simulink model "cardio_v3"  (Simulink 7.4)
settings: Solver=ode45  StartTime=0.0  StopTime=100  RelTol=1e-3
settings Model: Creator=hp  LastModifiedBy=MXKana
settings DebuggingCC: SaveWithParameterizedLinksMsg=none

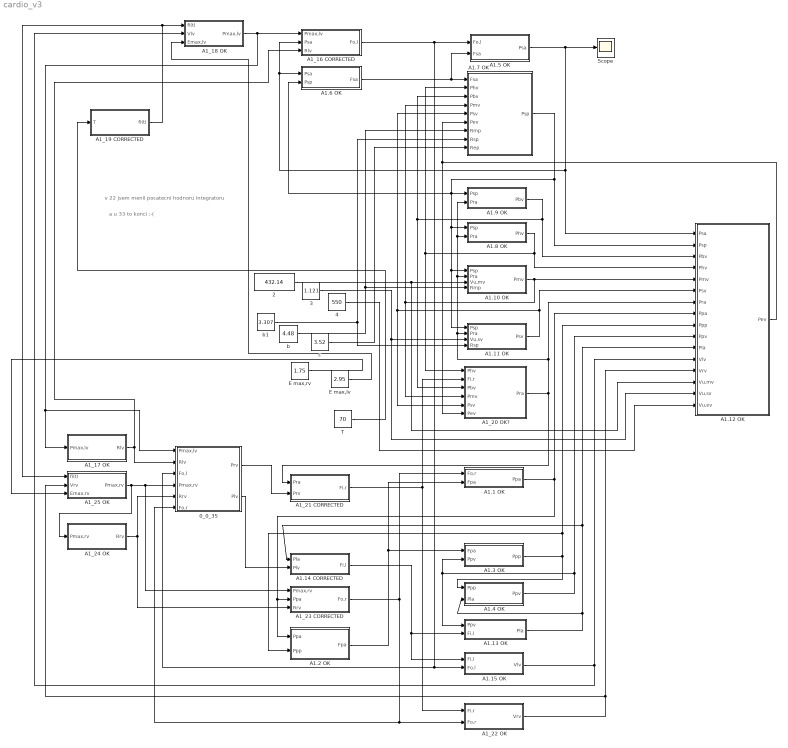
== system cardio_v3 ==
  note: v 22 jsem menil pocatecni hodnoru integratoru
  note: a u 33 to konci :-(
  0_0_35 : Subsystem
  2 : Constant  Value=432.14  OutDataType=sfix(16)  OutScaling=2^0
  3 : Constant  Value=1.121  OutDataType=sfix(16)  OutScaling=2^0
  4 : Constant  Value=550  OutDataType=sfix(16)  OutScaling=2^0
  A1.1 OK : Subsystem
  A1.10 OK : Subsystem
  A1.11 OK : Subsystem
  A1.12 OK : Subsystem
  A1.13 OK : Subsystem
  A1.14 CORRECTED : Subsystem
  A1.15 OK : Subsystem
  A1.2 OK : Subsystem
  A1.3 OK : Subsystem
  A1.4 OK : Subsystem
  A1.5 OK : Subsystem
  A1.6 OK : Subsystem
  A1.7 OK : Subsystem
  A1.8 OK : Subsystem
  A1.9 OK : Subsystem
  A1_16 CORRECTED : Subsystem
  A1_17 OK : Subsystem
  A1_18 OK : Subsystem
  A1_19 CORRECTED : Subsystem
  A1_20 OK? : Subsystem
  A1_21 CORRECTED : Subsystem
  A1_22 OK : Subsystem
  A1_23 CORRECTED : Subsystem
  A1_24 OK : Subsystem
  A1_25 OK : Subsystem
  "E max,lv " : Constant  Value=2.95  OutDataType=sfix(16)  OutScaling=2^0
  "E max,rv " : Constant  Value=1.75  OutDataType=sfix(16)  OutScaling=2^0
  Scope : Scope
  "T " : Constant  Value=70  OutDataType=sfix(16)  OutScaling=2^0
  b : Constant  Value=4.48  OutDataType=sfix(16)  OutScaling=2^0
  b1 : Constant  Value=3.307  OutDataType=sfix(16)  OutScaling=2^0
  c : Constant  Value=3.52  OutDataType=sfix(16)  OutScaling=2^0
  wires:
  A1.10 OK/1(Pmv) -> A1.12 OK/5(Pmv), A1.7 OK/4(Pmv), A1_20 OK?/4(Pmv)
  A1.11 OK/1(Psv) -> A1.12 OK/6(Psv), A1.7 OK/5(Psv), A1_20 OK?/5(Psv)
  A1.3 OK/1(Ppp) -> A1.4 OK/1(Ppp), A1.12 OK/9(Ppp), A1.2 OK/2(Ppp)
  A1.15 OK/1(Vlv) -> A1.12 OK/12(Vlv), A1_18 OK/2(Vlv)
  A1.4 OK/1(Ppv) -> A1.12 OK/10(Ppv), A1.3 OK/2(Ppv), A1.13 OK/1(Ppv)
  A1.13 OK/1(Pla) -> A1.4 OK/2(Pla), A1.12 OK/11(Pla), A1.14 CORRECTED/1(Pla)
  A1.8 OK/1(Phv) -> A1.12 OK/4(Phv), A1_20 OK?/1(Phv), A1.7 OK/2(Phv)
  A1.9 OK/1(Pbv) -> A1.12 OK/3(Pbv), A1.7 OK/3(Pbv), A1_20 OK?/3(Pbv)
  A1.7 OK/1(Psp) -> A1.12 OK/2(Psp), A1.9 OK/1(Psp), A1.8 OK/1(Psp), A1.10 OK/1(Psp), A1.11 OK/1(Psp), A1.6 OK/2(Psp)
  A1.5 OK/1(Psa) -> A1.12 OK/1(Psa), A1.6 OK/1(Psa), A1_16 CORRECTED/2(Psa), Scope/1
  A1_20 OK?/1(Pra) -> A1.12 OK/7(Pra), A1.10 OK/2(Pra), A1.8 OK/2(Pra), A1.9 OK/2(Pra), A1.11 OK/2(Pra), A1_21 CORRECTED/1(Pra)
  A1.1 OK/1(Ppa) -> A1.12 OK/8(Ppa), A1.2 OK/1(Ppa), A1_23 CORRECTED/2(Ppa)
  A1_22 OK/1(Vrv) -> A1.12 OK/13(Vrv), A1_25 OK/2(Vrv)
  A1_16 CORRECTED/1(Fo,l) -> A1.5 OK/1(Fo,l), A1.15 OK/2(Fo,l), 0_0_35/3(Fo,l)
  A1.6 OK/1(Fsa) -> A1.7 OK/1(Fsa), A1.5 OK/2(Fsa)
  A1.12 OK/1(Pev) -> A1.7 OK/6(Pev), A1_20 OK?/6(Pev)
  2/1 -> A1.10 OK/3(Vu,mv), A1.12 OK/14(Vu,mv)
  3/1 -> A1.11 OK/3(Vu,sv), A1.12 OK/15(Vu,sv)
  A1_21 CORRECTED/1(Fi,r) -> A1_20 OK?/2(Fi,r), A1_22 OK/1(Fi,r)
  A1.14 CORRECTED/1(Fi,l) -> A1.15 OK/1(Fi,l), A1.13 OK/2(Fi,l)
  A1_23 CORRECTED/1(Fo,r) -> A1.1 OK/1(Fo,r), A1_22 OK/2(Fo,r), 0_0_35/6(Fo,r)
  A1.2 OK/1(Fpa) -> A1.3 OK/1(Fpa), A1.1 OK/2(Fpa)
  A1_18 OK/1(Pmax,lv) -> A1_16 CORRECTED/1(Pmax,lv), A1_17 OK/1(Pmax,lv), 0_0_35/1(Pmax,lv)
  0_0_35/1(Prv) -> A1_21 CORRECTED/2(Prv)
  0_0_35/2(Plv) -> A1.14 CORRECTED/2(Plv)
  A1_25 OK/1(Pmax,rv) -> A1_24 OK/1(Pmax,rv), 0_0_35/4(Pmax,rv), A1_23 CORRECTED/1(Pmax,rv)
  A1_24 OK/1(Rrv) -> 0_0_35/5(Rrv), A1_23 CORRECTED/3(Rrv)
  A1_17 OK/1(Rlv) -> 0_0_35/2(Rlv), A1_16 CORRECTED/3(Rlv)
  A1_19 CORRECTED/1(fi(t)) -> A1_18 OK/1(fi(t)), A1_25 OK/1(fi(t))
  "T "/1 -> A1_19 CORRECTED/1(T)
  b1/1 -> A1.7 OK/8(Rsp), A1.11 OK/4(Rsp)
  b/1 -> A1.7 OK/7(Rmp), A1.10 OK/4(Rmp)
  c/1 -> A1.7 OK/9(Rep)
  "E max,lv "/1 -> A1_18 OK/3(Emax,lv)
  "E max,rv "/1 -> A1_25 OK/3(Emax,rv)
  4/1 -> A1.12 OK/16(Vu,ev)

== system cardio_v3/0_0_35 ==
  Pmax,lv : Inport  OutDataType=fixdt(1, 16)  OutScaling=2^0
  Rlv : Inport  Port=2  OutDataType=fixdt(1, 16)  OutScaling=2^0
  Fo,l : Inport  Port=3  OutDataType=fixdt(1, 16)  OutScaling=2^0
  Pmax,rv : Inport  Port=4  OutDataType=fixdt(1, 16)  OutScaling=2^0
  Rrv : Inport  Port=5  OutDataType=fixdt(1, 16)  OutScaling=2^0
  Fo,r : Inport  Port=6  OutDataType=fixdt(1, 16)  OutScaling=2^0
  Add : Sum  Inputs=+-  OutDataType=fixdt(1, 16)  OutScaling=2^-10
  Add1 : Sum  Inputs=+-  OutDataType=fixdt(1, 16)  OutScaling=2^-10
  Product : Product  OutDataType=fixdt(1, 16)  OutScaling=2^0  RndMeth=Zero
  Product1 : Product  OutDataType=fixdt(1, 16)  OutScaling=2^0  RndMeth=Zero
  Prv : Outport  OutDataType=fixdt(1, 16)  OutScaling=2^0
  Plv : Outport  Port=2  OutDataType=fixdt(1, 16)  OutScaling=2^0
  wires:
  Product1/1 -> Add1/2
  Fo,r/1 -> Product1/2
  Rrv/1 -> Product1/1
  Pmax,rv/1 -> Add1/1
  Product/1 -> Add/2
  Fo,l/1 -> Product/2
  Rlv/1 -> Product/1
  Pmax,lv/1 -> Add/1
  Add/1 -> Plv/1
  Add1/1 -> Prv/1

== system cardio_v3/A1.1 OK ==
  Fo,r : Inport  OutDataType=sfix(16)  OutScaling=2^0
  Fpa : Inport  Port=2  OutDataType=sfix(16)  OutScaling=2^0
  Add : Sum  Inputs=+-  OutDataType=sfix(16)  OutScaling=2^-10
  Constant : Constant  OutDataType=sfix(16)  OutScaling=2^0
  Cpa : Constant  Value=0.76  OutDataType=sfix(16)  OutScaling=2^0
  Divide : Product  Inputs=*/  OutDataType=sfix(16)  OutScaling=2^-10
  Integrator : Integrator
  Product : Product  OutDataType=sfix(16)  OutScaling=2^0  RndMeth=Zero
  Ppa : Outport  OutDataType=sfix(16)  OutScaling=2^0
  wires:
  Fpa/1 -> Add/2
  Fo,r/1 -> Add/1
  Cpa/1 -> Divide/2
  Integrator/1 -> Ppa/1
  Product/1 -> Integrator/1
  Add/1 -> Product/2
  Divide/1 -> Product/1
  Constant/1 -> Divide/1

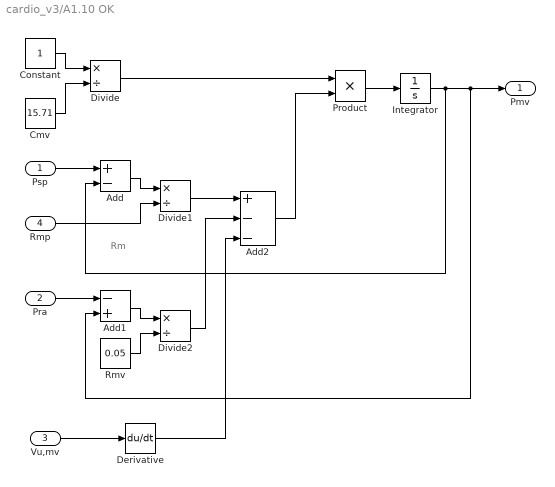
== system cardio_v3/A1.10 OK ==
  note: Rm
  Psp : Inport  OutDataType=sfix(16)  OutScaling=2^0
  Pra : Inport  Port=2  OutDataType=sfix(16)  OutScaling=2^0
  Vu,mv : Inport  Port=3  OutDataType=sfix(16)  OutScaling=2^0
  Rmp : Inport  Port=4  OutDataType=sfix(16)  OutScaling=2^0
  Add : Sum  Inputs=+-  OutDataType=sfix(16)  OutScaling=2^-10
  Add1 : Sum  Inputs=-+  OutDataType=sfix(16)  OutScaling=2^-10
  Add2 : Sum  Inputs=+--  OutDataType=sfix(16)  OutScaling=2^-10
  Cmv : Constant  Value=15.71  OutDataType=sfix(16)  OutScaling=2^0
  Constant : Constant  OutDataType=sfix(16)  OutScaling=2^0
  Derivative : Derivative
  Divide : Product  Inputs=*/  OutDataType=sfix(16)  OutScaling=2^-10
  Divide1 : Product  Inputs=*/  OutDataType=sfix(16)  OutScaling=2^-10
  Divide2 : Product  Inputs=*/  OutDataType=sfix(16)  OutScaling=2^-10
  Integrator : Integrator
  Product : Product  OutDataType=sfix(16)  OutScaling=2^0  RndMeth=Zero
  Rmv : Constant  Value=0.05  OutDataType=sfix(16)  OutScaling=2^0
  Pmv : Outport  OutDataType=sfix(16)  OutScaling=2^0
  wires:
  Derivative/1 -> Add2/3
  Vu,mv/1 -> Derivative/1
  Add2/1 -> Product/2
  Divide2/1 -> Add2/2
  Divide1/1 -> Add2/1
  Rmv/1 -> Divide2/2
  Add1/1 -> Divide2/1
  Rmp/1 -> Divide1/2
  Add/1 -> Divide1/1
  Pra/1 -> Add1/1
  Psp/1 -> Add/1
  Integrator/1 -> Add1/2, Pmv/1, Add/2
  Product/1 -> Integrator/1
  Divide/1 -> Product/1
  Cmv/1 -> Divide/2
  Constant/1 -> Divide/1

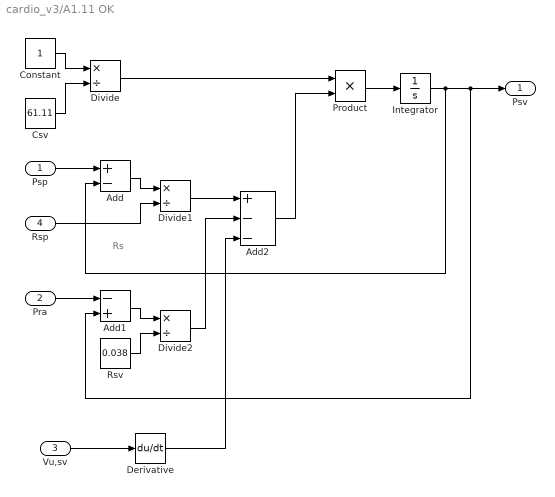
== system cardio_v3/A1.11 OK ==
  note: Rs
  Psp : Inport  OutDataType=sfix(16)  OutScaling=2^0
  Pra : Inport  Port=2  OutDataType=sfix(16)  OutScaling=2^0
  Vu,sv : Inport  Port=3  OutDataType=sfix(16)  OutScaling=2^0
  Rsp : Inport  Port=4  OutDataType=sfix(16)  OutScaling=2^0
  Add : Sum  Inputs=+-  OutDataType=sfix(16)  OutScaling=2^-10
  Add1 : Sum  Inputs=-+  OutDataType=sfix(16)  OutScaling=2^-10
  Add2 : Sum  Inputs=+--  OutDataType=sfix(16)  OutScaling=2^-10
  Constant : Constant  OutDataType=sfix(16)  OutScaling=2^0
  Csv : Constant  Value=61.11  OutDataType=sfix(16)  OutScaling=2^0
  Derivative : Derivative
  Divide : Product  Inputs=*/  OutDataType=sfix(16)  OutScaling=2^-10
  Divide1 : Product  Inputs=*/  OutDataType=sfix(16)  OutScaling=2^-10
  Divide2 : Product  Inputs=*/  OutDataType=sfix(16)  OutScaling=2^-10
  Integrator : Integrator
  Product : Product  OutDataType=sfix(16)  OutScaling=2^0  RndMeth=Zero
  Rsv : Constant  Value=0.038  OutDataType=sfix(16)  OutScaling=2^0
  Psv : Outport  OutDataType=sfix(16)  OutScaling=2^0
  wires:
  Derivative/1 -> Add2/3
  Vu,sv/1 -> Derivative/1
  Add2/1 -> Product/2
  Divide2/1 -> Add2/2
  Divide1/1 -> Add2/1
  Rsv/1 -> Divide2/2
  Add1/1 -> Divide2/1
  Rsp/1 -> Divide1/2
  Add/1 -> Divide1/1
  Pra/1 -> Add1/1
  Psp/1 -> Add/1
  Integrator/1 -> Add1/2, Psv/1, Add/2
  Product/1 -> Integrator/1
  Divide/1 -> Product/1
  Csv/1 -> Divide/2
  Constant/1 -> Divide/1

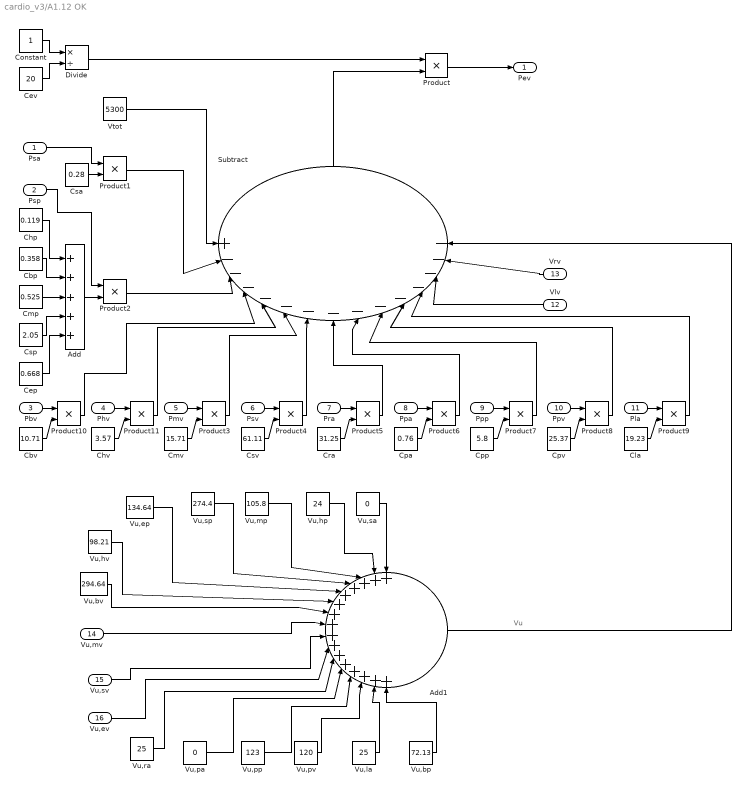
== system cardio_v3/A1.12 OK ==
  note: Vu
  Psa : Inport  OutDataType=sfix(16)  OutScaling=2^0
  Psp : Inport  Port=2  OutDataType=sfix(16)  OutScaling=2^0
  Pbv : Inport  Port=3  OutDataType=sfix(16)  OutScaling=2^0
  Phv : Inport  Port=4  OutDataType=sfix(16)  OutScaling=2^0
  Pmv : Inport  Port=5  OutDataType=sfix(16)  OutScaling=2^0
  Psv : Inport  Port=6  OutDataType=sfix(16)  OutScaling=2^0
  Pra : Inport  Port=7  OutDataType=sfix(16)  OutScaling=2^0
  Ppa : Inport  Port=8  OutDataType=sfix(16)  OutScaling=2^0
  Ppp : Inport  Port=9  OutDataType=sfix(16)  OutScaling=2^0
  Ppv : Inport  Port=10  OutDataType=sfix(16)  OutScaling=2^0
  Pla : Inport  Port=11  OutDataType=sfix(16)  OutScaling=2^0
  Vlv : Inport  Port=12  OutDataType=sfix(16)  OutScaling=2^0
  Vrv : Inport  Port=13  OutDataType=sfix(16)  OutScaling=2^0
  Vu,mv : Inport  Port=14  OutDataType=sfix(16)  OutScaling=2^0
  Vu,sv : Inport  Port=15  OutDataType=sfix(16)  OutScaling=2^0
  Vu,ev : Inport  Port=16  OutDataType=sfix(16)  OutScaling=2^0
  Add : Sum  Inputs=+++++  OutDataType=sfix(16)  OutScaling=2^-10
  Add1 : Sum  Inputs=++++++++++++++++  OutDataType=sfix(16)  OutScaling=2^-10
  Cbp : Constant  Value=0.358  OutDataType=sfix(16)  OutScaling=2^0
  Cbv : Constant  Value=10.71  OutDataType=sfix(16)  OutScaling=2^0
  Cep : Constant  Value=0.668  OutDataType=sfix(16)  OutScaling=2^0
  Cev : Constant  Value=20  OutDataType=sfix(16)  OutScaling=2^0
  Chp : Constant  Value=0.119  OutDataType=sfix(16)  OutScaling=2^0
  Chv : Constant  Value=3.57  OutDataType=sfix(16)  OutScaling=2^0
  Cla : Constant  Value=19.23  OutDataType=sfix(16)  OutScaling=2^0
  Cmp : Constant  Value=0.525  OutDataType=sfix(16)  OutScaling=2^0
  Cmv : Constant  Value=15.71  OutDataType=sfix(16)  OutScaling=2^0
  Constant : Constant  OutDataType=sfix(16)  OutScaling=2^0
  Cpa : Constant  Value=0.76  OutDataType=sfix(16)  OutScaling=2^0
  Cpp : Constant  Value=5.8  OutDataType=sfix(16)  OutScaling=2^0
  Cpv : Constant  Value=25.37  OutDataType=sfix(16)  OutScaling=2^0
  Cra : Constant  Value=31.25  OutDataType=sfix(16)  OutScaling=2^0
  Csa : Constant  Value=0.28  OutDataType=sfix(16)  OutScaling=2^0
  Csp : Constant  Value=2.05  OutDataType=sfix(16)  OutScaling=2^0
  Csv : Constant  Value=61.11  OutDataType=sfix(16)  OutScaling=2^0
  Divide : Product  Inputs=*/  OutDataType=sfix(16)  OutScaling=2^-10
  Product{,1..11} (12 alike) : Product  OutDataType=sfix(16)  OutScaling=2^0  RndMeth=Zero
  Subtract : Sum  Inputs=+--------------  OutDataType=sfix(16)  OutScaling=2^-10
  Vtot : Constant  Value=5300  OutDataType=sfix(16)  OutScaling=2^0
  Vu,bp : Constant  Value=72.13  OutDataType=sfix(16)  OutScaling=2^0
  Vu,bv : Constant  Value=294.64  OutDataType=sfix(16)  OutScaling=2^0
  Vu,ep : Constant  Value=134.64  OutDataType=sfix(16)  OutScaling=2^0
  Vu,hp : Constant  Value=24  OutDataType=sfix(16)  OutScaling=2^0
  Vu,hv : Constant  Value=98.21  OutDataType=sfix(16)  OutScaling=2^0
  Vu,la : Constant  Value=25  OutDataType=sfix(16)  OutScaling=2^0
  Vu,mp : Constant  Value=105.8  OutDataType=sfix(16)  OutScaling=2^0
  Vu,pa : Constant  Value=0  OutDataType=sfix(16)  OutScaling=2^0
  Vu,pp : Constant  Value=123  OutDataType=sfix(16)  OutScaling=2^0
  Vu,pv : Constant  Value=120  OutDataType=sfix(16)  OutScaling=2^0
  Vu,ra : Constant  Value=25  OutDataType=sfix(16)  OutScaling=2^0
  Vu,sa : Constant  Value=0  OutDataType=sfix(16)  OutScaling=2^0
  Vu,sp : Constant  Value=274.4  OutDataType=sfix(16)  OutScaling=2^0
  Pev : Outport  OutDataType=sfix(16)  OutScaling=2^0
  wires:
  Add1/1 -> Subtract/15
  Vu,sa/1 -> Add1/1
  Vu,hp/1 -> Add1/2
  Vu,mp/1 -> Add1/3
  Vu,sp/1 -> Add1/4
  Vu,ep/1 -> Add1/5
  Vu,hv/1 -> Add1/6
  Vu,bv/1 -> Add1/7
  Vu,mv/1 -> Add1/8
  Vu,sv/1 -> Add1/9
  Vu,ev/1 -> Add1/10
  Vu,ra/1 -> Add1/11
  Vu,pa/1 -> Add1/12
  Vu,pp/1 -> Add1/13
  Vu,pv/1 -> Add1/14
  Vu,la/1 -> Add1/15
  Vu,bp/1 -> Add1/16
  Subtract/1 -> Product/2
  Vrv/1 -> Subtract/14
  Vlv/1 -> Subtract/13
  Product3/1 -> Subtract/6
  Product2/1 -> Subtract/3
  Product1/1 -> Subtract/2
  Vtot/1 -> Subtract/1
  Product10/1 -> Subtract/4
  Product11/1 -> Subtract/5
  Chv/1 -> Product11/2
  Phv/1 -> Product11/1
  Cbv/1 -> Product10/2
  Pbv/1 -> Product10/1
  Product9/1 -> Subtract/12
  Product8/1 -> Subtract/11
  Product7/1 -> Subtract/10
  Product6/1 -> Subtract/9
  Product5/1 -> Subtract/8
  Product4/1 -> Subtract/7
  Cla/1 -> Product9/2
  Pla/1 -> Product9/1
  Cpv/1 -> Product8/2
  Ppv/1 -> Product8/1
  Cpp/1 -> Product7/2
  Ppp/1 -> Product7/1
  Cpa/1 -> Product6/2
  Ppa/1 -> Product6/1
  Cra/1 -> Product5/2
  Pra/1 -> Product5/1
  Csv/1 -> Product4/2
  Psv/1 -> Product4/1
  Cmv/1 -> Product3/2
  Pmv/1 -> Product3/1
  Psp/1 -> Product2/1
  Add/1 -> Product2/2
  Psa/1 -> Product1/1
  Csa/1 -> Product1/2
  Cep/1 -> Add/5
  Csp/1 -> Add/4
  Cmp/1 -> Add/3
  Cbp/1 -> Add/2
  Chp/1 -> Add/1
  Product/1 -> Pev/1
  Divide/1 -> Product/1
  Cev/1 -> Divide/2
  Constant/1 -> Divide/1

== system cardio_v3/A1.13 OK ==
  Ppv : Inport  OutDataType=sfix(16)  OutScaling=2^0
  Fi,l : Inport  Port=2  OutDataType=sfix(16)  OutScaling=2^0
  Add : Sum  Inputs=+-  OutDataType=sfix(16)  OutScaling=2^-10
  Cla : Constant  Value=19.23  OutDataType=sfix(16)  OutScaling=2^0
  Constant : Constant  OutDataType=sfix(16)  OutScaling=2^0
  Divide : Product  Inputs=*/  OutDataType=sfix(16)  OutScaling=2^-10
  Divide1 : Product  Inputs=*/  OutDataType=sfix(16)  OutScaling=2^-10
  Integrator : Integrator
  Product : Product  OutDataType=sfix(16)  OutScaling=2^0  RndMeth=Zero
  Rpv : Constant  Value=0.0056  OutDataType=sfix(16)  OutScaling=2^0
  Subtract : Sum  Inputs=+-  OutDataType=sfix(16)  OutScaling=2^-10
  Pla : Outport  OutDataType=sfix(16)  OutScaling=2^0
  wires:
  Add/1 -> Product/2
  Fi,l/1 -> Add/2
  Divide1/1 -> Add/1
  Rpv/1 -> Divide1/2
  Subtract/1 -> Divide1/1
  Ppv/1 -> Subtract/1
  Divide/1 -> Product/1
  Product/1 -> Integrator/1
  Cla/1 -> Divide/2
  Constant/1 -> Divide/1
  Integrator/1 -> Subtract/2, Pla/1

== system cardio_v3/A1.14 CORRECTED ==
  Pla : Inport  OutDataType=sfix(16)  OutScaling=2^0
  Plv : Inport  Port=2  OutDataType=sfix(16)  OutScaling=2^0
  Constant : Constant  Value=0  OutDataType=sfix(16)  OutScaling=2^0
  Divide : Product  Inputs=*/  OutDataType=sfix(16)  OutScaling=2^-10
  Gain : Gain  Gain=-1  ParameterDataType=fixdt(1, 16)  ParameterScaling=2^0  OutDataType=fixdt(1, 16)  OutScaling=2^0
  Rla : Constant  Value=0.0025  OutDataType=sfix(16)  OutScaling=2^0
  Subtract : Sum  Inputs=-+  OutDataType=sfix(16)  OutScaling=2^-10
  Switch : Switch
  Fi,l : Outport  OutDataType=sfix(16)  OutScaling=2^0
  wires:
  Divide/1 -> Switch/3
  Switch/1 -> Fi,l/1
  Subtract/1 -> Divide/1, Gain/1
  Pla/1 -> Subtract/2
  Rla/1 -> Divide/2
  Constant/1 -> Switch/1
  Plv/1 -> Subtract/1
  Gain/1 -> Switch/2

== system cardio_v3/A1.15 OK ==
  Fi,l : Inport  OutDataType=sfix(16)  OutScaling=2^0
  Fo,l : Inport  Port=2  OutDataType=sfix(16)  OutScaling=2^0
  Integrator : Integrator
  Subtract : Sum  Inputs=+-  OutDataType=sfix(16)  OutScaling=2^-10
  Vlv : Outport  OutDataType=sfix(16)  OutScaling=2^0
  wires:
  Integrator/1 -> Vlv/1
  Subtract/1 -> Integrator/1
  Fo,l/1 -> Subtract/2
  Fi,l/1 -> Subtract/1

== system cardio_v3/A1.2 OK ==
  Ppa : Inport  OutDataType=sfix(16)  OutScaling=2^0
  Ppp : Inport  Port=2  OutDataType=sfix(16)  OutScaling=2^0
  Add : Sum  Inputs=+--  OutDataType=sfix(16)  OutScaling=2^-10
  Constant : Constant  OutDataType=sfix(16)  OutScaling=2^0
  Divide : Product  Inputs=*/  OutDataType=sfix(16)  OutScaling=2^-10
  Integrator : Integrator
  Lpa : Constant  Value=0.00018  OutDataType=sfix(16)  OutScaling=2^0
  Product : Product  OutDataType=sfix(16)  OutScaling=2^0  RndMeth=Zero
  Product1 : Product  OutDataType=sfix(16)  OutScaling=2^0  RndMeth=Zero
  Rpa : Constant  Value=0.023  OutDataType=sfix(16)  OutScaling=2^0
  Fpa : Outport  OutDataType=sfix(16)  OutScaling=2^0
  wires:
  Integrator/1 -> Product1/2, Fpa/1
  Product/1 -> Integrator/1
  Add/1 -> Product/2
  Divide/1 -> Product/1
  Product1/1 -> Add/3
  Ppp/1 -> Add/2
  Ppa/1 -> Add/1
  Rpa/1 -> Product1/1
  Lpa/1 -> Divide/2
  Constant/1 -> Divide/1

== system cardio_v3/A1.3 OK ==
  Fpa : Inport  OutDataType=sfix(16)  OutScaling=2^0
  Ppv : Inport  Port=2  OutDataType=sfix(16)  OutScaling=2^0
  Add : Sum  Inputs=-+  OutDataType=sfix(16)  OutScaling=2^-10
  Add1 : Sum  Inputs=+-  OutDataType=sfix(16)  OutScaling=2^-10
  Constant : Constant  OutDataType=sfix(16)  OutScaling=2^0
  Cpp : Constant  Value=5.8  OutDataType=sfix(16)  OutScaling=2^0
  Divide : Product  Inputs=*/  OutDataType=sfix(16)  OutScaling=2^-10
  Divide1 : Product  Inputs=*/  OutDataType=sfix(16)  OutScaling=2^-10
  Integrator : Integrator
  Product : Product  OutDataType=sfix(16)  OutScaling=2^0  RndMeth=Zero
  Rpp : Constant  Value=0.0894  OutDataType=sfix(16)  OutScaling=2^0
  Ppp : Outport  OutDataType=sfix(16)  OutScaling=2^0
  wires:
  Product/1 -> Integrator/1
  Add1/1 -> Product/2
  Divide/1 -> Product/1
  Divide1/1 -> Add1/2
  Fpa/1 -> Add1/1
  Rpp/1 -> Divide1/2
  Add/1 -> Divide1/1
  Integrator/1 -> Add/2, Ppp/1
  Ppv/1 -> Add/1
  Cpp/1 -> Divide/2
  Constant/1 -> Divide/1

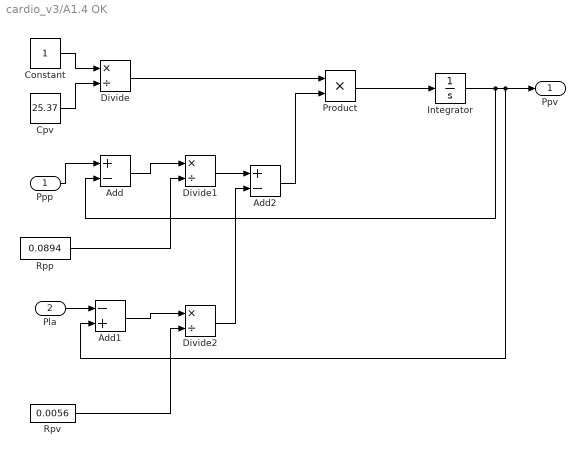
== system cardio_v3/A1.4 OK ==
  Ppp : Inport  OutDataType=sfix(16)  OutScaling=2^0
  Pla : Inport  Port=2  OutDataType=sfix(16)  OutScaling=2^0
  Add : Sum  Inputs=+-  OutDataType=sfix(16)  OutScaling=2^-10
  Add1 : Sum  Inputs=-+  OutDataType=sfix(16)  OutScaling=2^-10
  Add2 : Sum  Inputs=+-  OutDataType=sfix(16)  OutScaling=2^-10
  Constant : Constant  OutDataType=sfix(16)  OutScaling=2^0
  Cpv : Constant  Value=25.37  OutDataType=sfix(16)  OutScaling=2^0
  Divide : Product  Inputs=*/  OutDataType=sfix(16)  OutScaling=2^-10
  Divide1 : Product  Inputs=*/  OutDataType=sfix(16)  OutScaling=2^-10
  Divide2 : Product  Inputs=*/  OutDataType=sfix(16)  OutScaling=2^-10
  Integrator : Integrator
  Product : Product  OutDataType=sfix(16)  OutScaling=2^0  RndMeth=Zero
  Rpp : Constant  Value=0.0894  OutDataType=sfix(16)  OutScaling=2^0
  Rpv : Constant  Value=0.0056  OutDataType=sfix(16)  OutScaling=2^0
  Ppv : Outport  OutDataType=sfix(16)  OutScaling=2^0
  wires:
  Add2/1 -> Product/2
  Divide2/1 -> Add2/2
  Divide1/1 -> Add2/1
  Rpv/1 -> Divide2/2
  Rpp/1 -> Divide1/2
  Add/1 -> Divide1/1
  Add1/1 -> Divide2/1
  Pla/1 -> Add1/1
  Ppp/1 -> Add/1
  Integrator/1 -> Add1/2, Ppv/1, Add/2
  Product/1 -> Integrator/1
  Divide/1 -> Product/1
  Cpv/1 -> Divide/2
  Constant/1 -> Divide/1

== system cardio_v3/A1.5 OK ==
  Fo,l : Inport  OutDataType=sfix(16)  OutScaling=2^0
  Fsa : Inport  Port=2  OutDataType=sfix(16)  OutScaling=2^0
  Constant : Constant  OutDataType=sfix(16)  OutScaling=2^0
  Csa : Constant  Value=0.28  OutDataType=sfix(16)  OutScaling=2^0
  Divide : Product  Inputs=*/  OutDataType=sfix(16)  OutScaling=2^-10
  Integrator : Integrator
  Product : Product  OutDataType=sfix(16)  OutScaling=2^0  RndMeth=Zero
  Subtract : Sum  Inputs=+-  OutDataType=sfix(16)  OutScaling=2^-10
  Psa : Outport  OutDataType=sfix(16)  OutScaling=2^0
  wires:
  Constant/1 -> Divide/1
  Csa/1 -> Divide/2
  Integrator/1 -> Psa/1
  Product/1 -> Integrator/1
  Fsa/1 -> Subtract/2
  Fo,l/1 -> Subtract/1
  Subtract/1 -> Product/1
  Divide/1 -> Product/2

== system cardio_v3/A1.6 OK ==
  Psa : Inport  OutDataType=sfix(16)  OutScaling=2^0
  Psp : Inport  Port=2  OutDataType=sfix(16)  OutScaling=2^0
  Add : Sum  Inputs=+--  OutDataType=sfix(16)  OutScaling=2^-10
  Constant : Constant  OutDataType=sfix(16)  OutScaling=2^0
  Divide : Product  Inputs=*/  OutDataType=sfix(16)  OutScaling=2^-10
  Integrator : Integrator
  Lsa : Constant  Value=0.00022  OutDataType=sfix(16)  OutScaling=2^0
  Product : Product  OutDataType=sfix(16)  OutScaling=2^0  RndMeth=Zero
  Product1 : Product  OutDataType=sfix(16)  OutScaling=2^0  RndMeth=Zero
  Rsa : Constant  Value=0.06  OutDataType=sfix(16)  OutScaling=2^0
  Fsa : Outport  OutDataType=sfix(16)  OutScaling=2^0
  wires:
  Add/1 -> Product/2
  Product1/1 -> Add/3
  Psp/1 -> Add/2
  Psa/1 -> Add/1
  Rsa/1 -> Product1/1
  Integrator/1 -> Product1/2, Fsa/1
  Product/1 -> Integrator/1
  Divide/1 -> Product/1
  Lsa/1 -> Divide/2
  Constant/1 -> Divide/1

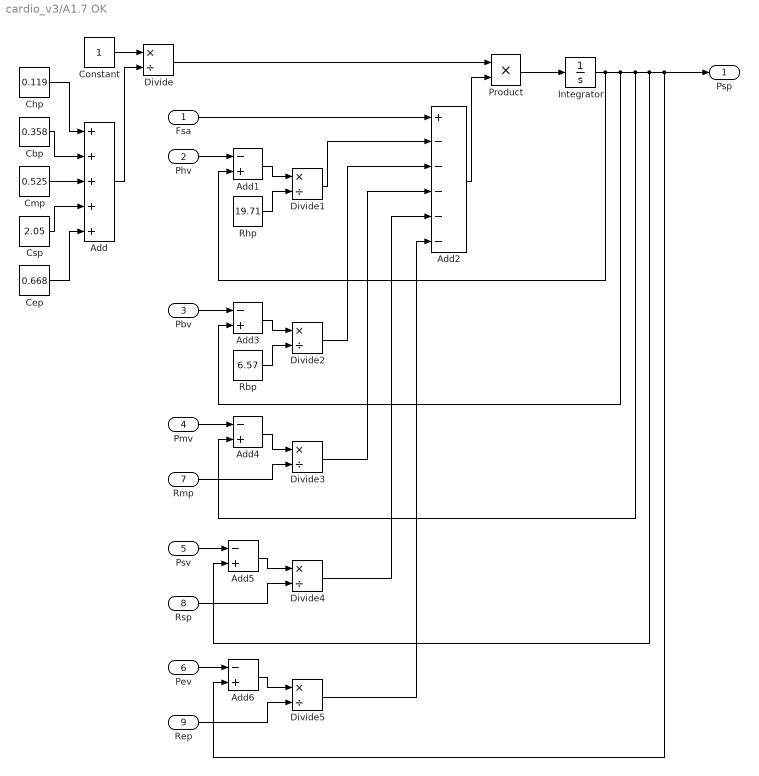
== system cardio_v3/A1.7 OK ==
  Fsa : Inport  OutDataType=sfix(16)  OutScaling=2^0
  Phv : Inport  Port=2  OutDataType=sfix(16)  OutScaling=2^0
  Pbv : Inport  Port=3  OutDataType=sfix(16)  OutScaling=2^0
  Pmv : Inport  Port=4  OutDataType=sfix(16)  OutScaling=2^0
  Psv : Inport  Port=5  OutDataType=sfix(16)  OutScaling=2^0
  Pev : Inport  Port=6  OutDataType=sfix(16)  OutScaling=2^0
  Rmp : Inport  Port=7  OutDataType=sfix(16)  OutScaling=2^0
  Rsp : Inport  Port=8  OutDataType=sfix(16)  OutScaling=2^0
  Rep : Inport  Port=9  OutDataType=sfix(16)  OutScaling=2^0
  Add : Sum  Inputs=+++++  OutDataType=sfix(16)  OutScaling=2^-10
  Add{1,3..6} (5 alike) : Sum  Inputs=-+  OutDataType=sfix(16)  OutScaling=2^-10
  Add2 : Sum  Inputs=+-----  OutDataType=sfix(16)  OutScaling=2^-10
  Cbp : Constant  Value=0.358  OutDataType=sfix(16)  OutScaling=2^0
  Cep : Constant  Value=0.668  OutDataType=sfix(16)  OutScaling=2^0
  Chp : Constant  Value=0.119  OutDataType=sfix(16)  OutScaling=2^0
  Cmp : Constant  Value=0.525  OutDataType=sfix(16)  OutScaling=2^0
  Constant : Constant  OutDataType=sfix(16)  OutScaling=2^0
  Csp : Constant  Value=2.05  OutDataType=sfix(16)  OutScaling=2^0
  Divide{,1..5} (6 alike) : Product  Inputs=*/  OutDataType=sfix(16)  OutScaling=2^-10
  Integrator : Integrator
  Product : Product  OutDataType=sfix(16)  OutScaling=2^0  RndMeth=Zero
  Rbp : Constant  Value=6.57  OutDataType=sfix(16)  OutScaling=2^0
  Rhp : Constant  Value=19.71  OutDataType=sfix(16)  OutScaling=2^0
  Psp : Outport  OutDataType=sfix(16)  OutScaling=2^0
  wires:
  Divide5/1 -> Add2/6
  Rep/1 -> Divide5/2
  Add6/1 -> Divide5/1
  Pev/1 -> Add6/1
  Divide4/1 -> Add2/5
  Rsp/1 -> Divide4/2
  Add5/1 -> Divide4/1
  Psv/1 -> Add5/1
  Divide3/1 -> Add2/4
  Rmp/1 -> Divide3/2
  Add4/1 -> Divide3/1
  Pmv/1 -> Add4/1
  Divide2/1 -> Add2/3
  Rbp/1 -> Divide2/2
  Add3/1 -> Divide2/1
  Pbv/1 -> Add3/1
  Divide1/1 -> Add2/2
  Fsa/1 -> Add2/1
  Add2/1 -> Product/2
  Rhp/1 -> Divide1/2
  Add1/1 -> Divide1/1
  Phv/1 -> Add1/1
  Divide/1 -> Product/1
  Add/1 -> Divide/2
  Constant/1 -> Divide/1
  Cep/1 -> Add/5
  Csp/1 -> Add/4
  Chp/1 -> Add/1
  Cbp/1 -> Add/2
  Cmp/1 -> Add/3
  Product/1 -> Integrator/1
  Integrator/1 -> Add6/2, Psp/1, Add5/2, Add4/2, Add3/2, Add1/2

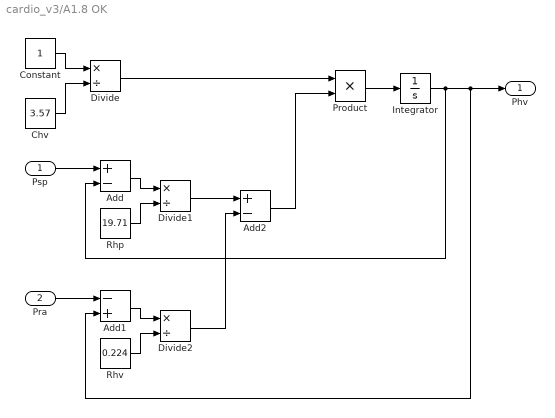
== system cardio_v3/A1.8 OK ==
  Psp : Inport  OutDataType=sfix(16)  OutScaling=2^0
  Pra : Inport  Port=2  OutDataType=sfix(16)  OutScaling=2^0
  Add : Sum  Inputs=+-  OutDataType=sfix(16)  OutScaling=2^-10
  Add1 : Sum  Inputs=-+  OutDataType=sfix(16)  OutScaling=2^-10
  Add2 : Sum  Inputs=+-  OutDataType=sfix(16)  OutScaling=2^-10
  Chv : Constant  Value=3.57  OutDataType=sfix(16)  OutScaling=2^0
  Constant : Constant  OutDataType=sfix(16)  OutScaling=2^0
  Divide : Product  Inputs=*/  OutDataType=sfix(16)  OutScaling=2^-10
  Divide1 : Product  Inputs=*/  OutDataType=sfix(16)  OutScaling=2^-10
  Divide2 : Product  Inputs=*/  OutDataType=sfix(16)  OutScaling=2^-10
  Integrator : Integrator
  Product : Product  OutDataType=sfix(16)  OutScaling=2^0  RndMeth=Zero
  Rhp : Constant  Value=19.71  OutDataType=sfix(16)  OutScaling=2^0
  Rhv : Constant  Value=0.224  OutDataType=sfix(16)  OutScaling=2^0
  Phv : Outport  OutDataType=sfix(16)  OutScaling=2^0
  wires:
  Add2/1 -> Product/2
  Divide2/1 -> Add2/2
  Divide1/1 -> Add2/1
  Rhv/1 -> Divide2/2
  Add1/1 -> Divide2/1
  Rhp/1 -> Divide1/2
  Add/1 -> Divide1/1
  Pra/1 -> Add1/1
  Psp/1 -> Add/1
  Integrator/1 -> Add1/2, Phv/1, Add/2
  Product/1 -> Integrator/1
  Divide/1 -> Product/1
  Chv/1 -> Divide/2
  Constant/1 -> Divide/1

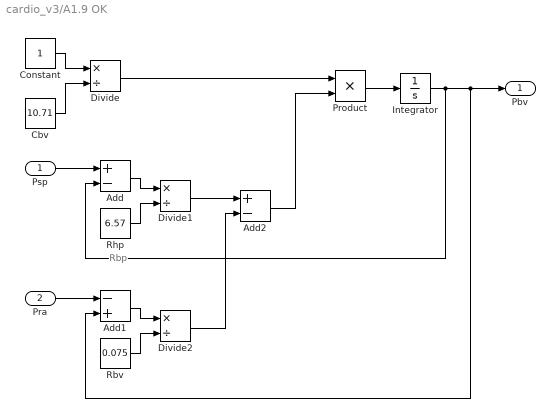
== system cardio_v3/A1.9 OK ==
  note: Rbp
  Psp : Inport  OutDataType=sfix(16)  OutScaling=2^0
  Pra : Inport  Port=2  OutDataType=sfix(16)  OutScaling=2^0
  Add : Sum  Inputs=+-  OutDataType=sfix(16)  OutScaling=2^-10
  Add1 : Sum  Inputs=-+  OutDataType=sfix(16)  OutScaling=2^-10
  Add2 : Sum  Inputs=+-  OutDataType=sfix(16)  OutScaling=2^-10
  Cbv : Constant  Value=10.71  OutDataType=sfix(16)  OutScaling=2^0
  Constant : Constant  OutDataType=sfix(16)  OutScaling=2^0
  Divide : Product  Inputs=*/  OutDataType=sfix(16)  OutScaling=2^-10
  Divide1 : Product  Inputs=*/  OutDataType=sfix(16)  OutScaling=2^-10
  Divide2 : Product  Inputs=*/  OutDataType=sfix(16)  OutScaling=2^-10
  Integrator : Integrator
  Product : Product  OutDataType=sfix(16)  OutScaling=2^0  RndMeth=Zero
  Rbv : Constant  Value=0.075  OutDataType=sfix(16)  OutScaling=2^0
  Rhp : Constant  Value=6.57  OutDataType=sfix(16)  OutScaling=2^0
  Pbv : Outport  OutDataType=sfix(16)  OutScaling=2^0
  wires:
  Add2/1 -> Product/2
  Divide2/1 -> Add2/2
  Divide1/1 -> Add2/1
  Rbv/1 -> Divide2/2
  Add1/1 -> Divide2/1
  Rhp/1 -> Divide1/2
  Add/1 -> Divide1/1
  Pra/1 -> Add1/1
  Psp/1 -> Add/1
  Integrator/1 -> Add1/2, Pbv/1, Add/2
  Product/1 -> Integrator/1
  Divide/1 -> Product/1
  Cbv/1 -> Divide/2
  Constant/1 -> Divide/1

== system cardio_v3/A1_16 CORRECTED ==
  Pmax,lv : Inport  OutDataType=sfix(16)  OutScaling=2^0
  Psa : Inport  Port=2  OutDataType=sfix(16)  OutScaling=2^0
  Rlv : Inport  Port=3  OutDataType=sfix(16)  OutScaling=2^0
  Constant : Constant  Value=0  OutDataType=sfix(16)  OutScaling=2^0
  Divide : Product  Inputs=*/  OutDataType=sfix(16)  OutScaling=2^-10
  Gain : Gain  Gain=-1  ParameterDataType=fixdt(1, 16)  ParameterScaling=2^0  OutDataType=fixdt(1, 16)  OutScaling=2^0
  Subtract : Sum  Inputs=+-  OutDataType=sfix(16)  OutScaling=2^-10
  Switch : Switch
  Fo,l : Outport  OutDataType=sfix(16)  OutScaling=2^0
  wires:
  Switch/1 -> Fo,l/1
  Divide/1 -> Switch/3
  Rlv/1 -> Divide/2
  Subtract/1 -> Divide/1, Gain/1
  Constant/1 -> Switch/1
  Psa/1 -> Subtract/2
  Pmax,lv/1 -> Subtract/1
  Gain/1 -> Switch/2

== system cardio_v3/A1_17 OK ==
  Pmax,lv : Inport  OutDataType=fixdt(1, 16)  OutScaling=2^0
  Product : Product  OutDataType=fixdt(1, 16)  OutScaling=2^0  RndMeth=Zero
  kR,lv : Constant  Value=0.000375  OutDataType=fixdt(1, 16)  OutScaling=2^0
  Rlv : Outport  OutDataType=fixdt(1, 16)  OutScaling=2^0
  wires:
  kR,lv/1 -> Product/2
  Pmax,lv/1 -> Product/1
  Product/1 -> Rlv/1

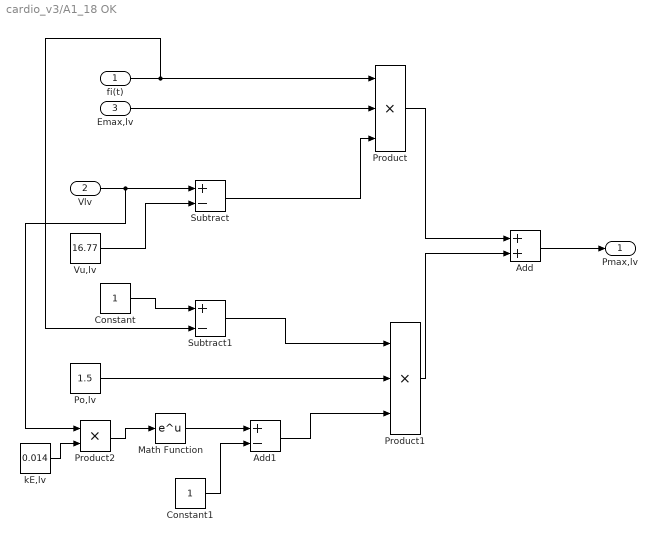
== system cardio_v3/A1_18 OK ==
  fi(t) : Inport  OutDataType=fixdt(1, 16)  OutScaling=2^0
  Vlv : Inport  Port=2  OutDataType=fixdt(1, 16)  OutScaling=2^0
  Emax,lv : Inport  Port=3  OutDataType=fixdt(1, 16)  OutScaling=2^0
  Add : Sum  OutDataType=fixdt(1, 16)  OutScaling=2^-10
  Add1 : Sum  Inputs=+-  OutDataType=fixdt(1, 16)  OutScaling=2^-10
  Constant : Constant  OutDataType=fixdt(1, 16)  OutScaling=2^0
  Constant1 : Constant  OutDataType=fixdt(1, 16)  OutScaling=2^0
  Math Function : Math  OutDataType=fixdt(1, 16)  OutScaling=2^0  SaturateOnIntegerOverflow=on
  Po,lv : Constant  Value=1.5  OutDataType=fixdt(1, 16)  OutScaling=2^0
  Product : Product  Inputs=3  OutDataType=fixdt(1, 16)  OutScaling=2^0  RndMeth=Zero
  Product1 : Product  Inputs=3  OutDataType=fixdt(1, 16)  OutScaling=2^0  RndMeth=Zero
  Product2 : Product  OutDataType=fixdt(1, 16)  OutScaling=2^0  RndMeth=Zero
  Subtract : Sum  Inputs=+-  OutDataType=fixdt(1, 16)  OutScaling=2^-10
  Subtract1 : Sum  Inputs=+-  OutDataType=fixdt(1, 16)  OutScaling=2^-10
  Vu,lv : Constant  Value=16.77  OutDataType=fixdt(1, 16)  OutScaling=2^0
  kE,lv : Constant  Value=0.014  OutDataType=fixdt(1, 16)  OutScaling=2^0
  Pmax,lv : Outport  OutDataType=fixdt(1, 16)  OutScaling=2^0
  wires:
  Math Function/1 -> Add1/1
  Product2/1 -> Math Function/1
  kE,lv/1 -> Product2/2
  Constant1/1 -> Add1/2
  Add1/1 -> Product1/3
  Po,lv/1 -> Product1/2
  Constant/1 -> Subtract1/1
  Subtract1/1 -> Product1/1
  Product1/1 -> Add/2
  Product/1 -> Add/1
  Add/1 -> Pmax,lv/1
  Subtract/1 -> Product/3
  Vu,lv/1 -> Subtract/2
  Vlv/1 -> Product2/1, Subtract/1
  Emax,lv/1 -> Product/2
  fi(t)/1 -> Subtract1/2, Product/1

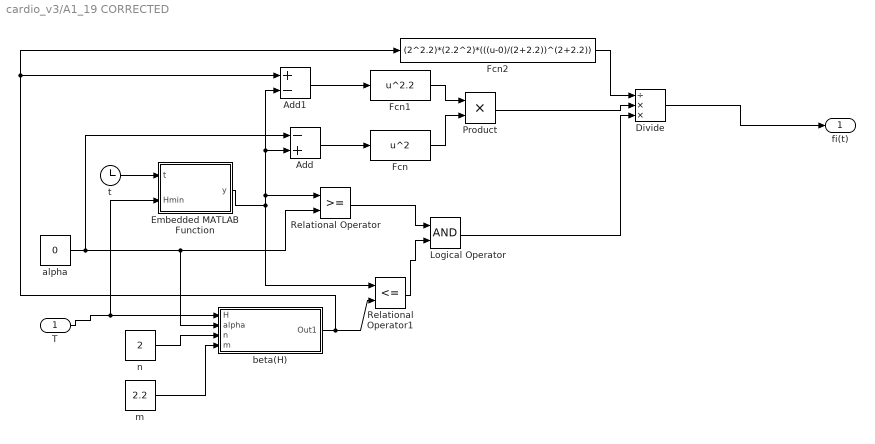
== system cardio_v3/A1_19 CORRECTED ==
  T : Inport  OutDataType=fixdt(1, 16)  OutScaling=2^0
  Add : Sum  Inputs=-+  OutDataType=sfix(16)  OutScaling=2^-10
  Add1 : Sum  Inputs=+-  OutDataType=sfix(16)  OutScaling=2^-10
  Divide : Product  Inputs=/**  OutDataType=sfix(16)  OutScaling=2^-10
  Embedded MATLAB Function : Stateflow chart
  Fcn : Fcn  Expr=u^2
  Fcn1 : Fcn  Expr=u^2.2
  Fcn2 : Fcn  Expr=(2^2.2)*(2.2^2)*(((u-0)/(2+2.2))^(2+2.2))
  Logical Operator : Logic  AllPortsSameDT=off  OutDataTypeMode=boolean  OutDataTypeStr=boolean
  Product : Product  OutDataType=sfix(16)  OutScaling=2^0  RndMeth=Zero
  Relational Operator : RelationalOperator  LogicOutDataTypeMode=boolean  OutDataTypeStr=boolean
  Relational Operator1 : RelationalOperator  Operator=<=  LogicOutDataTypeMode=boolean  OutDataTypeStr=boolean
  alpha : Constant  Value=0  OutDataType=sfix(16)  OutScaling=2^0
  beta(H) : Subsystem
  m : Constant  Value=2.2  OutDataType=sfix(16)  OutScaling=2^0
  n : Constant  Value=2  OutDataType=sfix(16)  OutScaling=2^0
  t : Clock
      settings: Decimation=10
  fi(t) : Outport  OutDataType=fixdt(1, 16)  OutScaling=2^0
  wires:
  alpha/1 -> Add/1, Relational Operator/2, beta(H)/2(alpha)
  Relational Operator/1 -> Logical Operator/1
  beta(H)/1(Out1) -> Relational Operator1/2, Add1/1, Fcn2/1
  Relational Operator1/1 -> Logical Operator/2
  Add/1 -> Fcn/1
  Add1/1 -> Fcn1/1
  Fcn1/1 -> Product/1
  Fcn/1 -> Product/2
  Product/1 -> Divide/2
  Fcn2/1 -> Divide/1
  Logical Operator/1 -> Divide/3
  T/1 -> beta(H)/1(H), Embedded MATLAB Function/2(Hmin)
  n/1 -> beta(H)/3(n)
  m/1 -> beta(H)/4(m)
  Divide/1 -> fi(t)/1
  Embedded MATLAB Function/1(y) -> Add1/2, Add/2, Relational Operator/1, Relational Operator1/1
  t/1 -> Embedded MATLAB Function/1(t)

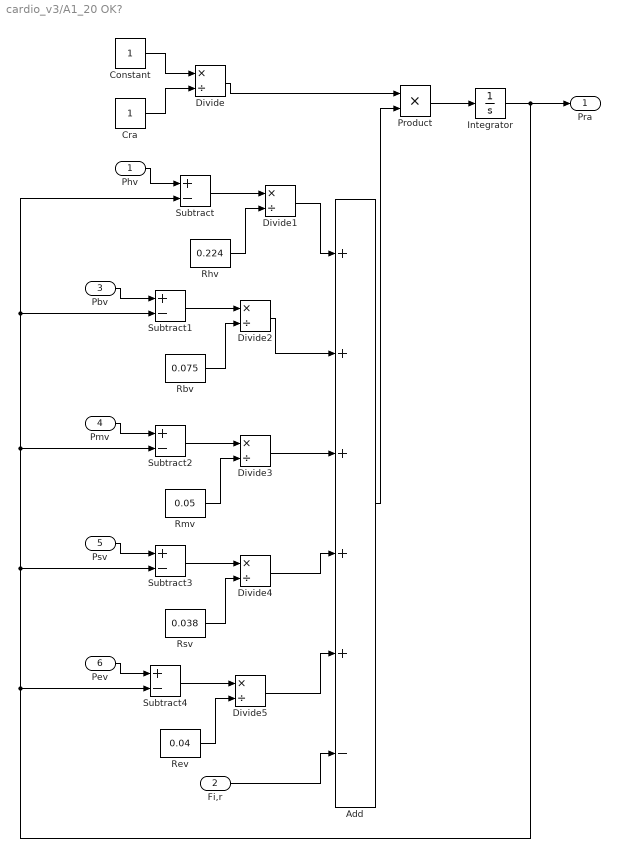
== system cardio_v3/A1_20 OK? ==
  Phv : Inport  OutDataType=sfix(16)  OutScaling=2^0
  Fi,r : Inport  Port=2  OutDataType=sfix(16)  OutScaling=2^0
  Pbv : Inport  Port=3  OutDataType=sfix(16)  OutScaling=2^0
  Pmv : Inport  Port=4  OutDataType=sfix(16)  OutScaling=2^0
  Psv : Inport  Port=5  OutDataType=sfix(16)  OutScaling=2^0
  Pev : Inport  Port=6  OutDataType=sfix(16)  OutScaling=2^0
  Add : Sum  Inputs=+++++-  OutDataType=sfix(16)  OutScaling=2^-10
  Constant : Constant  OutDataType=sfix(16)  OutScaling=2^0
  Cra : Constant  OutDataType=sfix(16)  OutScaling=2^0
  Divide{,1..5} (6 alike) : Product  Inputs=*/  OutDataType=sfix(16)  OutScaling=2^-10
  Integrator : Integrator
  Product : Product  OutDataType=sfix(16)  OutScaling=2^0  RndMeth=Zero
  Rbv : Constant  Value=0.075  OutDataType=sfix(16)  OutScaling=2^0
  Rev : Constant  Value=0.04  OutDataType=sfix(16)  OutScaling=2^0
  Rhv : Constant  Value=0.224  OutDataType=sfix(16)  OutScaling=2^0
  Rmv : Constant  Value=0.05  OutDataType=sfix(16)  OutScaling=2^0
  Rsv : Constant  Value=0.038  OutDataType=sfix(16)  OutScaling=2^0
  Subtract{,1..4} (5 alike) : Sum  Inputs=+-  OutDataType=sfix(16)  OutScaling=2^-10
  Pra : Outport  OutDataType=sfix(16)  OutScaling=2^0
  wires:
  Divide5/1 -> Add/5
  Rev/1 -> Divide5/2
  Subtract4/1 -> Divide5/1
  Pev/1 -> Subtract4/1
  Divide4/1 -> Add/4
  Rsv/1 -> Divide4/2
  Subtract3/1 -> Divide4/1
  Psv/1 -> Subtract3/1
  Divide3/1 -> Add/3
  Rmv/1 -> Divide3/2
  Subtract2/1 -> Divide3/1
  Pmv/1 -> Subtract2/1
  Divide2/1 -> Add/2
  Rbv/1 -> Divide2/2
  Subtract1/1 -> Divide2/1
  Pbv/1 -> Subtract1/1
  Fi,r/1 -> Add/6
  Add/1 -> Product/2
  Divide1/1 -> Add/1
  Rhv/1 -> Divide1/2
  Subtract/1 -> Divide1/1
  Phv/1 -> Subtract/1
  Divide/1 -> Product/1
  Product/1 -> Integrator/1
  Cra/1 -> Divide/2
  Constant/1 -> Divide/1
  Integrator/1 -> Subtract4/2, Subtract3/2, Subtract2/2, Subtract1/2, Subtract/2, Pra/1

== system cardio_v3/A1_21 CORRECTED ==
  Pra : Inport  OutDataType=sfix(16)  OutScaling=2^0
  Prv : Inport  Port=2  OutDataType=sfix(16)  OutScaling=2^0
  Constant : Constant  Value=0  OutDataType=sfix(16)  OutScaling=2^0
  Divide : Product  Inputs=*/  OutDataType=sfix(16)  OutScaling=2^-10
  Rra : Constant  Value=0.0025  OutDataType=sfix(16)  OutScaling=2^0
  Subtract : Sum  Inputs=+-  OutDataType=sfix(16)  OutScaling=2^-10
  Switch : Switch  Criteria=u2 > Threshold
  Fi,r : Outport  OutDataType=sfix(16)  OutScaling=2^0
  wires:
  Constant/1 -> Switch/3
  Divide/1 -> Switch/1
  Rra/1 -> Divide/2
  Subtract/1 -> Divide/1, Switch/2
  Prv/1 -> Subtract/2
  Pra/1 -> Subtract/1
  Switch/1 -> Fi,r/1

== system cardio_v3/A1_22 OK ==
  Fi,r : Inport  OutDataType=sfix(16)  OutScaling=2^0
  Fo,r : Inport  Port=2  OutDataType=sfix(16)  OutScaling=2^0
  Integrator : Integrator  InitialCondition=0.1
  Subtract : Sum  Inputs=+-  OutDataType=sfix(16)  OutScaling=2^-10
  Vrv : Outport  OutDataType=sfix(16)  OutScaling=2^0
  wires:
  Integrator/1 -> Vrv/1
  Subtract/1 -> Integrator/1
  Fo,r/1 -> Subtract/2
  Fi,r/1 -> Subtract/1

== system cardio_v3/A1_23 CORRECTED ==
  Pmax,rv : Inport  OutDataType=sfix(16)  OutScaling=2^0
  Ppa : Inport  Port=2  OutDataType=sfix(16)  OutScaling=2^0
  Rrv : Inport  Port=3  OutDataType=sfix(16)  OutScaling=2^0
  Constant : Constant  Value=0  OutDataType=sfix(16)  OutScaling=2^0
  Divide : Product  Inputs=*/  OutDataType=sfix(16)  OutScaling=2^-10
  Subtract : Sum  Inputs=+-  OutDataType=sfix(16)  OutScaling=2^-10
  Switch : Switch  Criteria=u2 > Threshold
  Fo,r : Outport  OutDataType=sfix(16)  OutScaling=2^0
  wires:
  Constant/1 -> Switch/3
  Divide/1 -> Switch/1
  Switch/1 -> Fo,r/1
  Rrv/1 -> Divide/2
  Subtract/1 -> Divide/1, Switch/2
  Ppa/1 -> Subtract/2
  Pmax,rv/1 -> Subtract/1

== system cardio_v3/A1_24 OK ==
  Pmax,rv : Inport  OutDataType=fixdt(1, 16)  OutScaling=2^0
  Product : Product  OutDataType=fixdt(1, 16)  OutScaling=2^0  RndMeth=Zero
  kR,rv : Constant  Value=0.0014  OutDataType=fixdt(1, 16)  OutScaling=2^0
  Rrv : Outport  OutDataType=fixdt(1, 16)  OutScaling=2^0
  wires:
  kR,rv/1 -> Product/2
  Pmax,rv/1 -> Product/1
  Product/1 -> Rrv/1

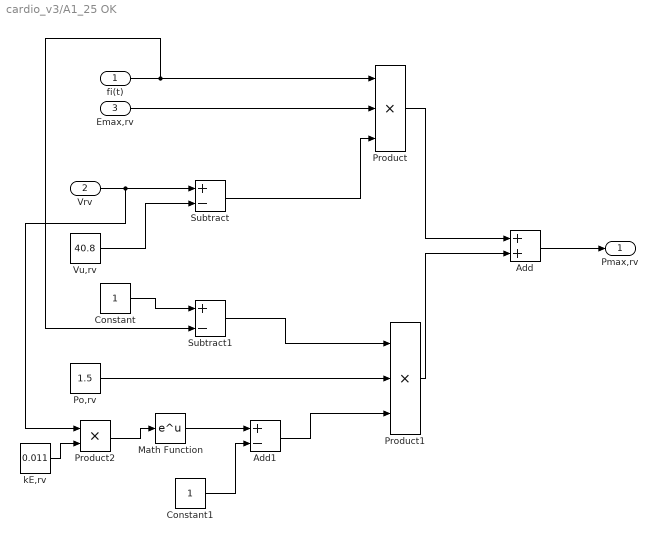
== system cardio_v3/A1_25 OK ==
  fi(t) : Inport  OutDataType=fixdt(1, 16)  OutScaling=2^0
  Vrv : Inport  Port=2  OutDataType=fixdt(1, 16)  OutScaling=2^0
  Emax,rv : Inport  Port=3  OutDataType=fixdt(1, 16)  OutScaling=2^0
  Add : Sum  OutDataType=fixdt(1, 16)  OutScaling=2^-10
  Add1 : Sum  Inputs=+-  OutDataType=fixdt(1, 16)  OutScaling=2^-10
  Constant : Constant  OutDataType=fixdt(1, 16)  OutScaling=2^0
  Constant1 : Constant  OutDataType=fixdt(1, 16)  OutScaling=2^0
  Math Function : Math  OutDataType=fixdt(1, 16)  OutScaling=2^0  SaturateOnIntegerOverflow=on
  Po,rv : Constant  Value=1.5  OutDataType=fixdt(1, 16)  OutScaling=2^0
  Product : Product  Inputs=3  OutDataType=fixdt(1, 16)  OutScaling=2^0  RndMeth=Zero
  Product1 : Product  Inputs=3  OutDataType=fixdt(1, 16)  OutScaling=2^0  RndMeth=Zero
  Product2 : Product  OutDataType=fixdt(1, 16)  OutScaling=2^0  RndMeth=Zero
  Subtract : Sum  Inputs=+-  OutDataType=fixdt(1, 16)  OutScaling=2^-10
  Subtract1 : Sum  Inputs=+-  OutDataType=fixdt(1, 16)  OutScaling=2^-10
  Vu,rv : Constant  Value=40.8  OutDataType=fixdt(1, 16)  OutScaling=2^0
  kE,rv : Constant  Value=0.011  OutDataType=fixdt(1, 16)  OutScaling=2^0
  Pmax,rv : Outport  OutDataType=fixdt(1, 16)  OutScaling=2^0
  wires:
  Math Function/1 -> Add1/1
  Product2/1 -> Math Function/1
  kE,rv/1 -> Product2/2
  Constant1/1 -> Add1/2
  Add1/1 -> Product1/3
  Po,rv/1 -> Product1/2
  Constant/1 -> Subtract1/1
  Subtract1/1 -> Product1/1
  Product1/1 -> Add/2
  Product/1 -> Add/1
  Add/1 -> Pmax,rv/1
  Subtract/1 -> Product/3
  Vu,rv/1 -> Subtract/2
  Vrv/1 -> Product2/1, Subtract/1
  Emax,rv/1 -> Product/2
  fi(t)/1 -> Subtract1/2, Product/1

== system cardio_v3/A1_19 CORRECTED/beta(H) ==
  H : Inport  OutDataType=sfix(16)  OutScaling=2^0
  alpha : Inport  Port=2  OutDataType=sfix(16)  OutScaling=2^0
  n : Inport  Port=3  OutDataType=sfix(16)  OutScaling=2^0
  m : Inport  Port=4  OutDataType=sfix(16)  OutScaling=2^0
  Add : Sum  OutDataType=sfix(16)  OutScaling=2^-10
  Add1 : Sum  Inputs=+-  OutDataType=sfix(16)  OutScaling=2^-10
  Divide : Product  Inputs=**/  OutDataType=sfix(16)  OutScaling=2^-10
  Product : Product  OutDataType=sfix(16)  OutScaling=2^0  RndMeth=Zero
  t p(H) : Fcn  Expr=0.1859+(1/(u^9.9+1))*(0.2799-0.1859)
  Out1 : Outport  OutDataType=sfix(16)  OutScaling=2^0
  wires:
  n/1 -> Add/1, Divide/3
  m/1 -> Add/2, Divide/2
  Add/1 -> Product/2
  t p(H)/1 -> Product/1
  H/1 -> t p(H)/1
  Product/1 -> Add1/1
  alpha/1 -> Divide/1
  Divide/1 -> Add1/2
  Add1/1 -> Out1/1

== matlab function A1_19 CORRECTED/Embedded MATLAB Function ==
  data: t input double; y output double; Hmin input double
function y = fcn(t,Hmin)
% This block supports an embeddable subset of the MATLAB language.
% See the help menu for details. 

y = mod(t,60/Hmin);
